simulink model "uzay_vektor"  (R2019b)
settings: Solver=ode1  StartTime=0.0  StopTime=0.02  FixedStep=1e-6  RelTol=1e-3
values from neighbouring files (symbols this model uses):
  m = 0.90    (= 0.9)    [uzay_vektor_parametreleri.m]
  Ts = 1/5000    (= 0.0002)    [uzay_vektor_parametreleri.m]
  Vdc = 250    [uzay_vektor_parametreleri.m]
  w = 2*pi*50    (= 314.159265359)    [uzay_vektor_parametreleri.m]
libraries: powerlib x20, simulink x12
settings Model: Creator=Monster  LastModifiedBy=Monster

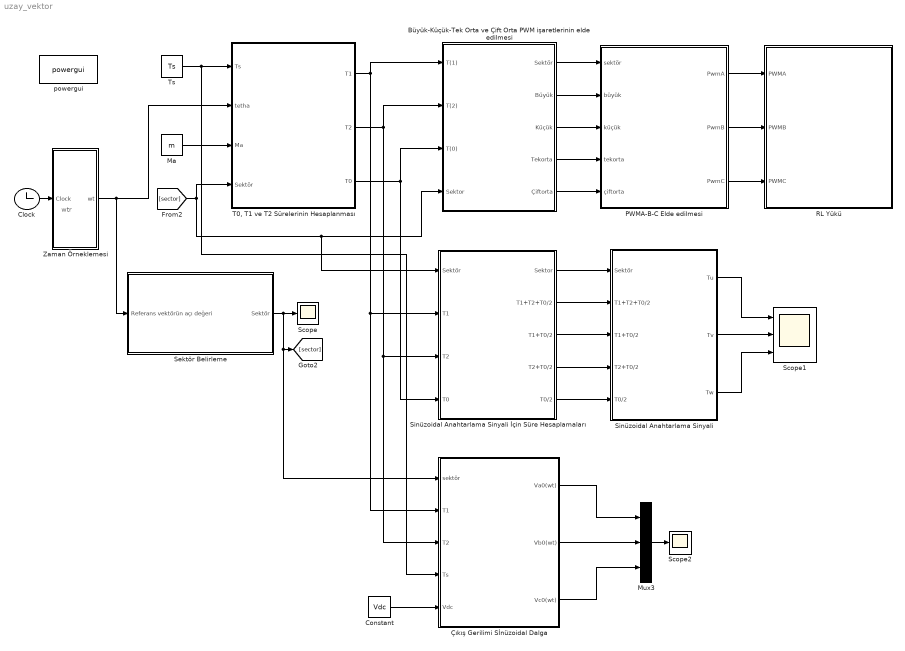
== system uzay_vektor ==
  note: wtr
  " Büyük-Küçük-Tek Orta ve Çift Orta PWM işaretlerinin elde edilmesi" : Subsystem
  " Clock" : Clock
  " Ma" : Constant  Value=m
  " PWMA-B-C Elde edilmesi" : Subsystem
  " RL Yükü" : Subsystem
  " Sektör Belirleme" : Subsystem
  " Sinüzoidal Anahtarlama Sinyali" : Subsystem
  " Sinüzoidal Anahtarlama Sinyali İçin Süre Hesaplamaları" : Subsystem
  " T0, T1 ve T2 Sürelerinin Hesaplanması" : Subsystem
  " Ts" : Constant  Value=Ts
  " Zaman Örneklemesi" : Subsystem
  " Çıkış Gerilimi Sİnüzoidal Dalga" : Subsystem
  Constant : Constant  Value=Vdc
  Mux3 : Mux  Inputs=3
  Scope : Scope
  Scope1 : Scope  NumInputPorts=3
  Scope2 : Scope
  "powergui " : powerlib/powergui  Priority=1  SimulationMode=Continuous  SampleTime=50e-6  frequency=60  Iterations=50  frequencyindice=0  Pbase=100e6  ErrMax=1e-4  UnitsV=kV  UnitsW=MW  buscounter=0  FunctionMessages=off  echomessages=off  EnableUseOfTLC=off  CurrentSourceSwitches=off  DisableSnubberDevices=off  DisableRonSwitches=off  DisableVfSwitches=off  DisplayEquations=off  AutomaticDiscreteSolvers=off  SolverType=Tustin/Backward Euler (TBE)  Interpol=off  ExternalGateDelay=off  methode=off  Ts=100  x0status=blocks  SPID=on  SwTol=0  HookPort=off  NonlinearTolerance=1e-4  nMaxIteration=100  ContinueOnMaxIteration=off  RestoreLinks=warning  ResistiveCurrentMeasurement=off  Frange=[0:2:500]  Ylog=off  Xlog=on  ShowGrid=off  save=off  variable=ZData  structure=0  ZoomFFT=off  StartTime=0.0  cycles=1  DisplayStyle=1  fundamental=60  FreqAxis=off  MaxFrequency=1000  frequencyindicesteady=1  RmsSteady=1  display=off
      settings: SourceProductName=Simscape Electrical
  wires:
  " Sektör Belirleme"/1(Sektör) -> " Çıkış Gerilimi Sİnüzoidal Dalga"/1("sektör "), [sector], Scope/1
  " Ts"/1 -> " Çıkış Gerilimi Sİnüzoidal Dalga"/4(Ts), " T0, T1 ve T2 Sürelerinin Hesaplanması"/1(Ts)
  [sector] -> " Sinüzoidal Anahtarlama Sinyali İçin Süre Hesaplamaları"/1(Sektör), " Büyük-Küçük-Tek Orta ve Çift Orta PWM işaretlerinin elde edilmesi"/4("Sektor "), " T0, T1 ve T2 Sürelerinin Hesaplanması"/4(Sektör)
  " Zaman Örneklemesi"/1("wt ") -> " Sektör Belirleme"/1(" Referans vektörün açı değeri"), " T0, T1 ve T2 Sürelerinin Hesaplanması"/2(tetha)
  " Clock"/1 -> " Zaman Örneklemesi"/1(Clock)
  " Ma"/1 -> " T0, T1 ve T2 Sürelerinin Hesaplanması"/3(Ma)
  " Büyük-Küçük-Tek Orta ve Çift Orta PWM işaretlerinin elde edilmesi"/1(Sektör) -> " PWMA-B-C Elde edilmesi"/1(sektör)
  " Büyük-Küçük-Tek Orta ve Çift Orta PWM işaretlerinin elde edilmesi"/2(Büyük) -> " PWMA-B-C Elde edilmesi"/2(büyük)
  " Büyük-Küçük-Tek Orta ve Çift Orta PWM işaretlerinin elde edilmesi"/3(Küçük) -> " PWMA-B-C Elde edilmesi"/3(küçük)
  " Büyük-Küçük-Tek Orta ve Çift Orta PWM işaretlerinin elde edilmesi"/4(Tekorta) -> " PWMA-B-C Elde edilmesi"/4(tekorta)
  " Büyük-Küçük-Tek Orta ve Çift Orta PWM işaretlerinin elde edilmesi"/5(Çiftorta) -> " PWMA-B-C Elde edilmesi"/5(çiftorta)
  " T0, T1 ve T2 Sürelerinin Hesaplanması"/3(T0) -> " Büyük-Küçük-Tek Orta ve Çift Orta PWM işaretlerinin elde edilmesi"/3(T(0)), " Sinüzoidal Anahtarlama Sinyali İçin Süre Hesaplamaları"/4(T0)
  " T0, T1 ve T2 Sürelerinin Hesaplanması"/2(T2) -> " Çıkış Gerilimi Sİnüzoidal Dalga"/3(T2), " Sinüzoidal Anahtarlama Sinyali İçin Süre Hesaplamaları"/3(T2), " Büyük-Küçük-Tek Orta ve Çift Orta PWM işaretlerinin elde edilmesi"/2(T(2))
  " T0, T1 ve T2 Sürelerinin Hesaplanması"/1(T1) -> " Çıkış Gerilimi Sİnüzoidal Dalga"/2(T1), " Sinüzoidal Anahtarlama Sinyali İçin Süre Hesaplamaları"/2(T1), " Büyük-Küçük-Tek Orta ve Çift Orta PWM işaretlerinin elde edilmesi"/1(T(1))
  " Sinüzoidal Anahtarlama Sinyali İçin Süre Hesaplamaları"/1(Sektor) -> " Sinüzoidal Anahtarlama Sinyali"/1(" Sektör")
  " Sinüzoidal Anahtarlama Sinyali İçin Süre Hesaplamaları"/2(T1+T2+T0/2) -> " Sinüzoidal Anahtarlama Sinyali"/2(" T1+T2+T0/2")
  " Sinüzoidal Anahtarlama Sinyali İçin Süre Hesaplamaları"/3(T1+T0/2) -> " Sinüzoidal Anahtarlama Sinyali"/3(" T1+T0/2")
  " Sinüzoidal Anahtarlama Sinyali İçin Süre Hesaplamaları"/4(T2+T0/2) -> " Sinüzoidal Anahtarlama Sinyali"/4(" T2+T0/2")
  " Sinüzoidal Anahtarlama Sinyali İçin Süre Hesaplamaları"/5(T0/2) -> " Sinüzoidal Anahtarlama Sinyali"/5(" T0/2")
  " Sinüzoidal Anahtarlama Sinyali"/2(" Tv") -> Scope1/2
  " Sinüzoidal Anahtarlama Sinyali"/1(" Tu") -> Scope1/1
  " Sinüzoidal Anahtarlama Sinyali"/3(" Tw") -> Scope1/3
  " PWMA-B-C Elde edilmesi"/1("PwmA ") -> " RL Yükü"/1(PWMA)
  " PWMA-B-C Elde edilmesi"/2("PwmB ") -> " RL Yükü"/2(PWMB)
  " PWMA-B-C Elde edilmesi"/3(PwmC) -> " RL Yükü"/3(PWMC)
  Mux3/1 -> Scope2/1
  " Çıkış Gerilimi Sİnüzoidal Dalga"/3(Vc0(wt)) -> Mux3/3
  " Çıkış Gerilimi Sİnüzoidal Dalga"/1(Va0(wt)) -> Mux3/1
  " Çıkış Gerilimi Sİnüzoidal Dalga"/2(Vb0(wt)) -> Mux3/2
  Constant/1 -> " Çıkış Gerilimi Sİnüzoidal Dalga"/5(Vdc)

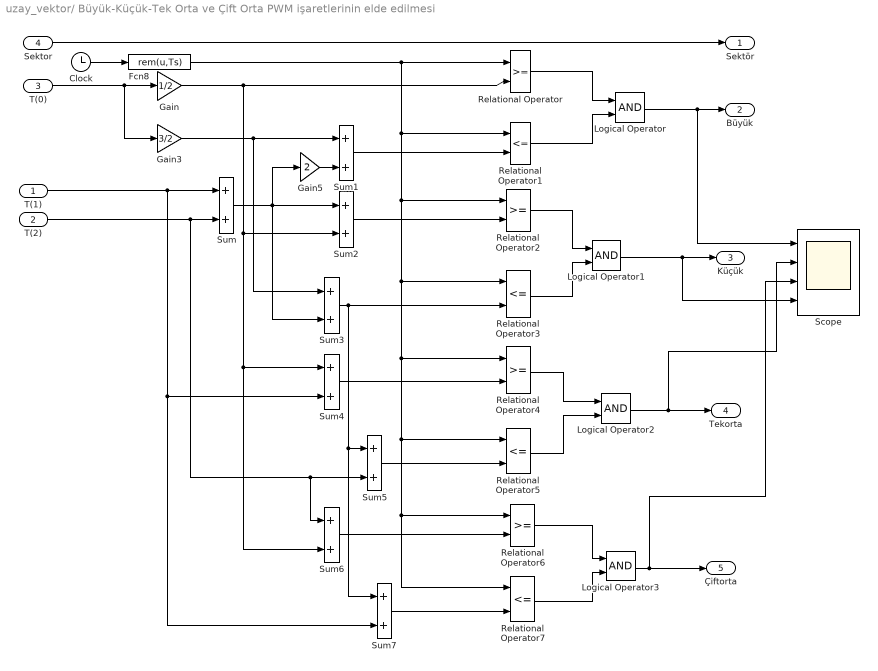
== system uzay_vektor/ Büyük-Küçük-Tek Orta ve Çift Orta PWM işaretlerinin elde edilmesi ==
  T(1) : Inport
  T(2) : Inport  Port=2
  T(0) : Inport  Port=3
  "Sektor " : Inport  Port=4
  Clock : Clock
  Fcn8 : Fcn  Expr=rem(u,Ts)
  Gain : Gain  Gain=1/2  SaturateOnIntegerOverflow=on  OutDataTypeStr=Inherit: Same as input  ParamDataTypeStr=Inherit: Same as input
  Gain3 : Gain  Gain=3/2  SaturateOnIntegerOverflow=on  OutDataTypeStr=Inherit: Same as input  ParamDataTypeStr=Inherit: Same as input
  Gain5 : Gain  Gain=2  SaturateOnIntegerOverflow=on  OutDataTypeStr=Inherit: Same as input  ParamDataTypeStr=Inherit: Same as input
  Logical Operator{,1..3} (4 alike) : Logic  AllPortsSameDT=off
  Relational Operator{,2,4,6} (4 alike) : RelationalOperator  RndMeth=Nearest
  Relational Operator{1,3,5,7} (4 alike) : RelationalOperator  Operator=<=  RndMeth=Nearest
  Scope : Scope  NumInputPorts=4
  Sum{,1..7} (8 alike) : Sum  SaturateOnIntegerOverflow=on
  Sektör : Outport
  Büyük : Outport  Port=2
  Küçük : Outport  Port=3
  Tekorta : Outport  Port=4
  Çiftorta : Outport  Port=5
  wires:
  Sum7/1 -> Relational Operator7/2
  Sum6/1 -> Relational Operator6/2
  Sum5/1 -> Relational Operator5/2
  Sum2/1 -> Relational Operator2/2
  Gain5/1 -> Sum1/2
  Gain3/1 -> Sum3/1, Sum1/1
  Sum/1 -> Sum3/2, Sum2/1, Gain5/1
  Clock/1 -> Fcn8/1
  Fcn8/1 -> Relational Operator/1, Relational Operator1/1, Relational Operator2/1, Relational Operator3/1, Relational Operator4/1, Relational Operator5/1, Relational Operator6/1, Relational Operator7/1
  T(0)/1 -> Gain3/1, Gain/1
  Gain/1 -> Relational Operator/2, Sum6/2, Sum4/1, Sum2/2
  T(1)/1 -> Sum7/2, Sum4/2, Sum/1
  T(2)/1 -> Sum6/1, Sum5/2, Sum/2
  Sum1/1 -> Relational Operator1/2
  Relational Operator/1 -> Logical Operator/1
  Relational Operator1/1 -> Logical Operator/2
  Logical Operator/1 -> Büyük/1, Scope/1
  Relational Operator2/1 -> Logical Operator1/1
  Relational Operator3/1 -> Logical Operator1/2
  Sum3/1 -> Sum7/1, Sum5/1, Relational Operator3/2
  Logical Operator1/1 -> Küçük/1, Scope/4
  Sum4/1 -> Relational Operator4/2
  Relational Operator4/1 -> Logical Operator2/1
  Relational Operator5/1 -> Logical Operator2/2
  Logical Operator2/1 -> Tekorta/1, Scope/2
  Relational Operator6/1 -> Logical Operator3/1
  Relational Operator7/1 -> Logical Operator3/2
  Logical Operator3/1 -> Çiftorta/1, Scope/3
  "Sektor "/1 -> Sektör/1

== system uzay_vektor/ PWMA-B-C Elde edilmesi ==
  sektör : Inport
  büyük : Inport  Port=2
  küçük : Inport  Port=3
  tekorta : Inport  Port=4
  çiftorta : Inport  Port=5
  PWMA-B-C : Scope  NumInputPorts=3
  Subsystem1 : Subsystem
  Subsystem2 : Subsystem
  Subsystem3 : Subsystem
  "PwmA " : Outport
  "PwmB " : Outport  Port=2
  PwmC : Outport  Port=3
  wires:
  sektör/1 -> Subsystem3/1(sektör), Subsystem1/1(sektör), Subsystem2/1(sektör)
  büyük/1 -> Subsystem3/2(Büyük), Subsystem1/2(Büyük), Subsystem2/2(Büyük)
  küçük/1 -> Subsystem3/3(Küçük), Subsystem1/3(Küçük), Subsystem2/3(Küçük)
  tekorta/1 -> Subsystem3/4(Tekorta), Subsystem1/4(Tekorta), Subsystem2/4(Tekorta)
  çiftorta/1 -> Subsystem3/5(çiftorta), Subsystem1/5(çiftorta), Subsystem2/5(çiftorta)
  Subsystem2/1(pwma) -> "PwmA "/1, PWMA-B-C/1
  Subsystem3/1(pwmc) -> PWMA-B-C/3, PwmC/1
  Subsystem1/1(pwmb) -> "PwmB "/1, PWMA-B-C/2

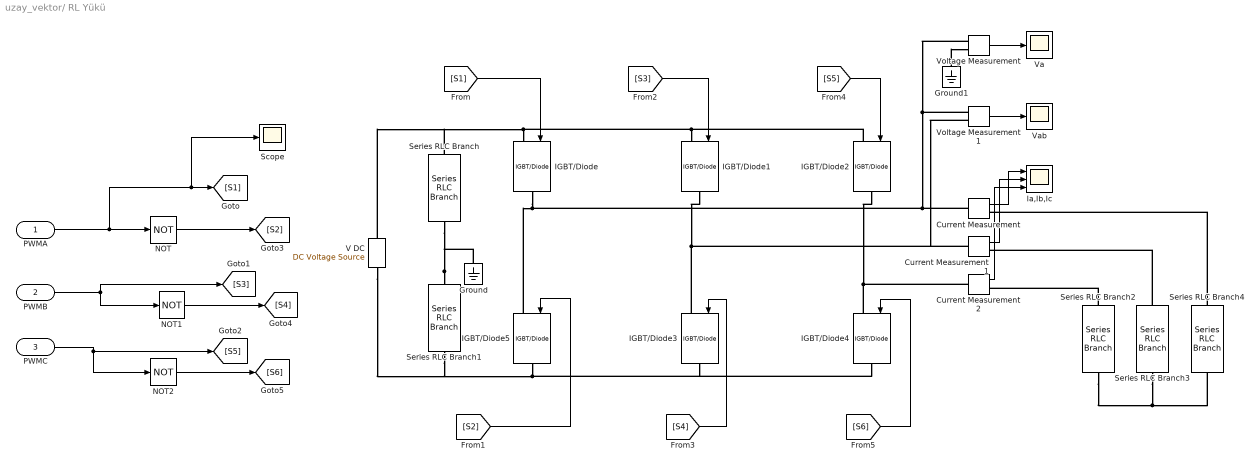
== system uzay_vektor/ RL Yükü ==
  PWMA : Inport
  PWMB : Inport  Port=2
  PWMC : Inport  Port=3
  " V DC" : powerlib/Electrical Sources/DC Voltage Source  Amplitude=Vdc  Measurements=None
      settings: SourceProductName=Simscape Electrical
  Current Measurement : powerlib/Measurements/Current Measurement  PhasorSimulation=off  OutputType=Complex  PSBequivalent=0
      settings: SourceProductName=Simscape Electrical
  Current Measurement1 : powerlib/Measurements/Current Measurement  PhasorSimulation=off  OutputType=Complex  PSBequivalent=0
      settings: SourceProductName=Simscape Electrical
  Current Measurement2 : powerlib/Measurements/Current Measurement  PhasorSimulation=off  OutputType=Complex  PSBequivalent=0
      settings: SourceProductName=Simscape Electrical
  Ground : powerlib/Elements/Ground  LConnTagsString=a
      settings: SourceProductName=Simscape Electrical
  Ground1 : powerlib/Elements/Ground  LConnTagsString=a
      settings: SourceProductName=Simscape Electrical
  "IGBT/Diode " : powerlib/Power Electronics/IGBT//Diode  Ron=1e-3  Rs=1e5  Cs=inf  Measurements=off
      settings: SourceProductName=Simscape Electrical
  IGBT/Diode{1..5} (5 alike) : powerlib/Power Electronics/IGBT//Diode  Ron=1e-3  Rs=1e5  Cs=inf  Measurements=off
      settings: SourceProductName=Simscape Electrical
  Ia,Ib,Ic : Scope  NumInputPorts=3
  "NOT " : Logic  Operator=NOT  IconShape=distinctive  AllPortsSameDT=off  OutDataTypeStr=boolean
  NOT1 : Logic  Operator=NOT  IconShape=distinctive  AllPortsSameDT=off  OutDataTypeStr=boolean
  NOT2 : Logic  Operator=NOT  IconShape=distinctive  AllPortsSameDT=off  OutDataTypeStr=boolean
  Scope : Scope
  Series RLC Branch : powerlib/Elements/Series RLC Branch  LConnTagsString=__new0  RConnTagsString=__new0  BranchType=RC  Resistance=0.01  Inductance=5000e-6  SetiL0=off  InitialCurrent=0  Capacitance=5000e-6  Setx0=off  InitialVoltage=0  Measurements=None
      settings: SourceProductName=Simscape Electrical
  Series RLC Branch1 : powerlib/Elements/Series RLC Branch  LConnTagsString=__new0  RConnTagsString=__new0  BranchType=RC  Resistance=0.01  Inductance=5000e-6  SetiL0=off  InitialCurrent=0  Capacitance=5000e-6  Setx0=off  InitialVoltage=0  Measurements=None
      settings: SourceProductName=Simscape Electrical
  Series RLC Branch2 : powerlib/Elements/Series RLC Branch  LConnTagsString=__new0  RConnTagsString=__new0  BranchType=RL  Resistance=30  Inductance=30e-3  SetiL0=off  InitialCurrent=0  Capacitance=30e-3  Setx0=off  InitialVoltage=0  Measurements=None
      settings: SourceProductName=Simscape Electrical
  Series RLC Branch3 : powerlib/Elements/Series RLC Branch  LConnTagsString=__new0  RConnTagsString=__new0  BranchType=RL  Resistance=30  Inductance=30e-3  SetiL0=off  InitialCurrent=0  Capacitance=30e-3  Setx0=off  InitialVoltage=0  Measurements=None
      settings: SourceProductName=Simscape Electrical
  Series RLC Branch4 : powerlib/Elements/Series RLC Branch  LConnTagsString=__new0  RConnTagsString=__new0  BranchType=RL  Resistance=30  Inductance=30e-3  SetiL0=off  InitialCurrent=0  Capacitance=30e-3  Setx0=off  InitialVoltage=0  Measurements=None
      settings: SourceProductName=Simscape Electrical
  Va : Scope
  Vab : Scope
  Voltage Measurement : powerlib/Measurements/Voltage Measurement  PhasorSimulation=off  OutputType=Complex  PSBequivalent=0
      settings: SourceProductName=Simscape Electrical
  Voltage Measurement1 : powerlib/Measurements/Voltage Measurement  PhasorSimulation=off  OutputType=Complex  PSBequivalent=0
      settings: SourceProductName=Simscape Electrical
  wires:
  [S4] -> IGBT/Diode3/1
  Current Measurement2/1 -> Ia,Ib,Ic/3
  Current Measurement/1 -> Ia,Ib,Ic/1
  Current Measurement1/1 -> Ia,Ib,Ic/2
  Voltage Measurement1/1 -> Vab/1
  Voltage Measurement/1 -> Va/1
  PWMA/1 -> "NOT "/1, Scope/1, [S1]
  [S5] -> IGBT/Diode2/1
  "NOT "/1 -> [S2]
  NOT2/1 -> [S6]
  PWMC/1 -> NOT2/1, [S5]
  [S1] -> "IGBT/Diode "/1
  NOT1/1 -> [S4]
  [S3] -> IGBT/Diode1/1
  [S2] -> IGBT/Diode5/1
  [S6] -> IGBT/Diode4/1
  PWMB/1 -> NOT1/1, [S3]
  connections:
  Voltage Measurement1/LConn1 -- Current Measurement/LConn1 -- IGBT/Diode5/LConn1 -- "IGBT/Diode "/RConn1 -- Voltage Measurement/LConn1
  IGBT/Diode2/RConn1 -- Current Measurement2/LConn1 -- IGBT/Diode4/LConn1
  IGBT/Diode5/RConn1 -- " V DC"/LConn1 -- Series RLC Branch1/RConn1 -- IGBT/Diode4/RConn1 -- IGBT/Diode3/RConn1
  Series RLC Branch3/RConn1 -- Series RLC Branch2/RConn1 -- Series RLC Branch4/RConn1
  IGBT/Diode1/RConn1 -- Current Measurement1/LConn1 -- Voltage Measurement1/LConn2 -- IGBT/Diode3/LConn1
  Series RLC Branch1/LConn1 -- Ground/LConn1 -- Series RLC Branch/RConn1
  IGBT/Diode1/LConn1 -- " V DC"/RConn1 -- Series RLC Branch/LConn1 -- "IGBT/Diode "/LConn1 -- IGBT/Diode2/LConn1
  Series RLC Branch2/LConn1 -- Current Measurement2/RConn1
  Ground1/LConn1 -- Voltage Measurement/LConn2
  Series RLC Branch4/LConn1 -- Current Measurement/RConn1
  Series RLC Branch3/LConn1 -- Current Measurement1/RConn1

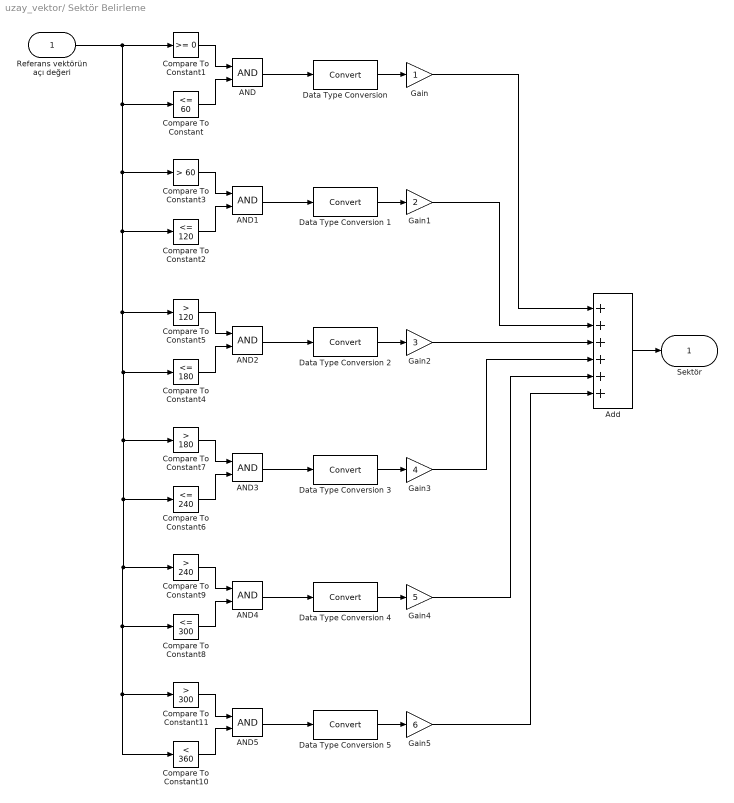
== system uzay_vektor/ Sektör Belirleme ==
  " Referans vektörün açı değeri" : Inport
  AND{,1..5} (6 alike) : Logic  AllPortsSameDT=off  OutDataTypeStr=boolean
  Add : Sum  Inputs=++++++
  Compare To Constant : simulink/Logic and Bit Operations/Compare To Constant  relop=<=  const=60  OutDataTypeStr=boolean
  Compare To Constant1 : simulink/Logic and Bit Operations/Compare To Constant  relop=>=  const=0  OutDataTypeStr=boolean
  Compare To Constant10 : simulink/Logic and Bit Operations/Compare To Constant  relop=<  const=360  OutDataTypeStr=boolean
  Compare To Constant11 : simulink/Logic and Bit Operations/Compare To Constant  relop=>  const=300  OutDataTypeStr=boolean
  Compare To Constant2 : simulink/Logic and Bit Operations/Compare To Constant  relop=<=  const=120  OutDataTypeStr=boolean
  Compare To Constant3 : simulink/Logic and Bit Operations/Compare To Constant  relop=>  const=60  OutDataTypeStr=boolean
  Compare To Constant4 : simulink/Logic and Bit Operations/Compare To Constant  relop=<=  const=180  OutDataTypeStr=boolean
  Compare To Constant5 : simulink/Logic and Bit Operations/Compare To Constant  relop=>  const=120  OutDataTypeStr=boolean
  Compare To Constant6 : simulink/Logic and Bit Operations/Compare To Constant  relop=<=  const=240  OutDataTypeStr=boolean
  Compare To Constant7 : simulink/Logic and Bit Operations/Compare To Constant  relop=>  const=180  OutDataTypeStr=boolean
  Compare To Constant8 : simulink/Logic and Bit Operations/Compare To Constant  relop=<=  const=300  OutDataTypeStr=boolean
  Compare To Constant9 : simulink/Logic and Bit Operations/Compare To Constant  relop=>  const=240  OutDataTypeStr=boolean
  Data Type Conversion {,1..5} (6 alike) : DataTypeConversion
  Gain : Gain
  Gain1 : Gain  Gain=2
  Gain2 : Gain  Gain=3
  Gain3 : Gain  Gain=4
  Gain4 : Gain  Gain=5
  Gain5 : Gain  Gain=6
  Sektör : Outport
  wires:
  Compare To Constant1/1 -> AND/1
  Compare To Constant/1 -> AND/2
  AND/1 -> "Data Type Conversion "/1
  "Data Type Conversion "/1 -> Gain/1
  Data Type Conversion 1/1 -> Gain1/1
  AND1/1 -> Data Type Conversion 1/1
  Compare To Constant2/1 -> AND1/2
  Compare To Constant3/1 -> AND1/1
  Compare To Constant7/1 -> AND3/1
  Compare To Constant6/1 -> AND3/2
  AND3/1 -> Data Type Conversion 3/1
  Data Type Conversion 3/1 -> Gain3/1
  Data Type Conversion 2/1 -> Gain2/1
  AND2/1 -> Data Type Conversion 2/1
  Compare To Constant4/1 -> AND2/2
  Compare To Constant5/1 -> AND2/1
  Compare To Constant9/1 -> AND4/1
  Compare To Constant8/1 -> AND4/2
  AND4/1 -> Data Type Conversion 4/1
  Data Type Conversion 4/1 -> Gain4/1
  Data Type Conversion 5/1 -> Gain5/1
  AND5/1 -> Data Type Conversion 5/1
  Compare To Constant10/1 -> AND5/2
  Compare To Constant11/1 -> AND5/1
  " Referans vektörün açı değeri"/1 -> Compare To Constant10/1, Compare To Constant11/1, Compare To Constant8/1, Compare To Constant9/1, Compare To Constant6/1, Compare To Constant7/1, Compare To Constant4/1, Compare To Constant5/1, Compare To Constant2/1, Compare To Constant3/1, Compare To Constant/1, Compare To Constant1/1
  Gain/1 -> Add/1
  Gain1/1 -> Add/2
  Gain2/1 -> Add/3
  Gain3/1 -> Add/4
  Gain4/1 -> Add/5
  Gain5/1 -> Add/6
  Add/1 -> Sektör/1

== system uzay_vektor/ Sinüzoidal Anahtarlama Sinyali ==
  " Sektör" : Inport
  " T1+T2+T0/2" : Inport  Port=2
  " T1+T0/2" : Inport  Port=3
  " T2+T0/2" : Inport  Port=4
  " T0/2" : Inport  Port=5
  S1 : MultiPortSwitch  DataPortOrder=Specify indices  Inputs=6  DataPortIndices={[1,6], 2,5,[3,4]}
  S3 : MultiPortSwitch  DataPortOrder=Specify indices  Inputs=6  DataPortIndices={ [2, 3], 4,1, [5, 6]}
  S5 : MultiPortSwitch  DataPortOrder=Specify indices  Inputs=6  DataPortIndices={ [4,5],6, 3, [1, 2]}
  " Tu" : Outport
  " Tv" : Outport  Port=2
  " Tw" : Outport  Port=3
  wires:
  S3/1 -> " Tv"/1
  S5/1 -> " Tw"/1
  S1/1 -> " Tu"/1
  " Sektör"/1 -> S5/1, S3/1, S1/1
  " T2+T0/2"/1 -> S1/4, S5/4, S3/4
  " T1+T0/2"/1 -> S1/3, S5/3, S3/3
  " T1+T2+T0/2"/1 -> S1/2, S5/2, S3/2
  " T0/2"/1 -> S1/5, S5/5, S3/5

== system uzay_vektor/ Sinüzoidal Anahtarlama Sinyali İçin Süre Hesaplamaları ==
  Sektör : Inport
  T1 : Inport  Port=2
  T2 : Inport  Port=3
  T0 : Inport  Port=4
  Add : Sum
  Add1 : Sum
  Gain : Gain  Gain=1/2
  TOPLAMA : Sum  Inputs=+++
  Sektor : Outport
  T1+T2+T0/2 : Outport  Port=2
  T1+T0/2 : Outport  Port=3
  T2+T0/2 : Outport  Port=4
  T0/2 : Outport  Port=5
  wires:
  T0/1 -> Gain/1
  T1/1 -> Add/1, TOPLAMA/1
  T2/1 -> TOPLAMA/2, Add1/1
  Gain/1 -> T0/2/1, Add1/2, Add/2, TOPLAMA/3
  TOPLAMA/1 -> T1+T2+T0/2/1
  Add/1 -> T1+T0/2/1
  Add1/1 -> T2+T0/2/1
  Sektör/1 -> Sektor/1

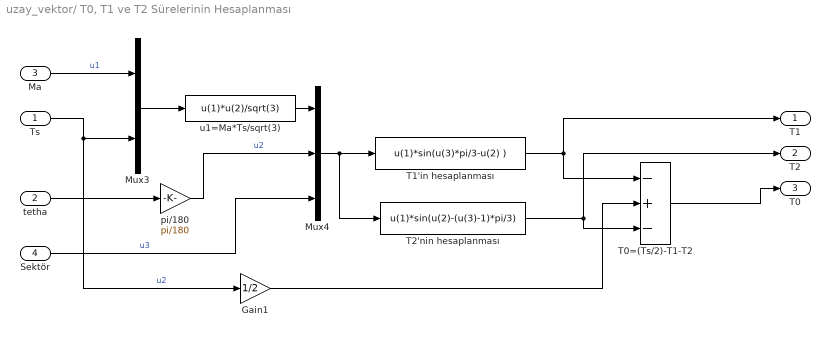
== system uzay_vektor/ T0, T1 ve T2 Sürelerinin Hesaplanması ==
  Ts : Inport
  tetha : Inport  Port=2
  Ma : Inport  Port=3
  Sektör : Inport  Port=4
  Gain1 : Gain  Gain=1/2
  Mux3 : Mux  Inputs=2
  Mux4 : Mux  Inputs=3
  T0=(Ts/2)-T1-T2 : Sum  Inputs=-+-
  T1'in hesaplanması : Fcn  Expr=u(1)*sin(u(3)*pi/3-u(2) )
  T2'nin hesaplanması : Fcn  Expr=u(1)*sin(u(2)-(u(3)-1)*pi/3)
  pi/180 : Gain  Gain=pi/180
  u1=Ma*Ts/sqrt(3) : Fcn  Expr=u(1)*u(2)/sqrt(3)
  T1 : Outport
  T2 : Outport  Port=2
  T0 : Outport  Port=3
  wires:
  T1'in hesaplanması/1 -> T0=(Ts/2)-T1-T2/1, T1/1
  T2'nin hesaplanması/1 -> T0=(Ts/2)-T1-T2/3, T2/1
  Mux3/1 -> u1=Ma*Ts/sqrt(3)/1
  Mux4/1 -> T2'nin hesaplanması/1, T1'in hesaplanması/1
  u1=Ma*Ts/sqrt(3)/1 -> Mux4/1
  Ts/1 -> Gain1/1, Mux3/2  "u2"
  Sektör/1 -> Mux4/3  "u3"
  Gain1/1 -> T0=(Ts/2)-T1-T2/2
  tetha/1 -> pi/180/1
  pi/180/1 -> Mux4/2  "u2"
  Ma/1 -> Mux3/1  "u1"
  T0=(Ts/2)-T1-T2/1 -> T0/1

== system uzay_vektor/ Zaman Örneklemesi ==
  Clock : Inport
  2*pi*50 : Constant  Value=w
  Constant2 : Constant  Value=2*pi
  Constant3 : Constant  Value=180/pi
  Math Function : Math  Operator=mod  SaturateOnIntegerOverflow=on
  Product1 : Product
  Product2 : Product  SaturateOnIntegerOverflow=on  OutDataTypeStr=Inherit: Same as first input
  "Scope " : Scope
  "Zero-Order Hold " : ZeroOrderHold  SampleTime=Ts
  "wt " : Outport
  wires:
  Product1/1 -> "Scope "/1, "wt "/1
  "Zero-Order Hold "/1 -> Product2/1
  2*pi*50/1 -> Product2/2
  Clock/1 -> "Zero-Order Hold "/1
  Constant3/1 -> Product1/2
  Constant2/1 -> Math Function/2
  Product2/1 -> Math Function/1
  Math Function/1 -> Product1/1

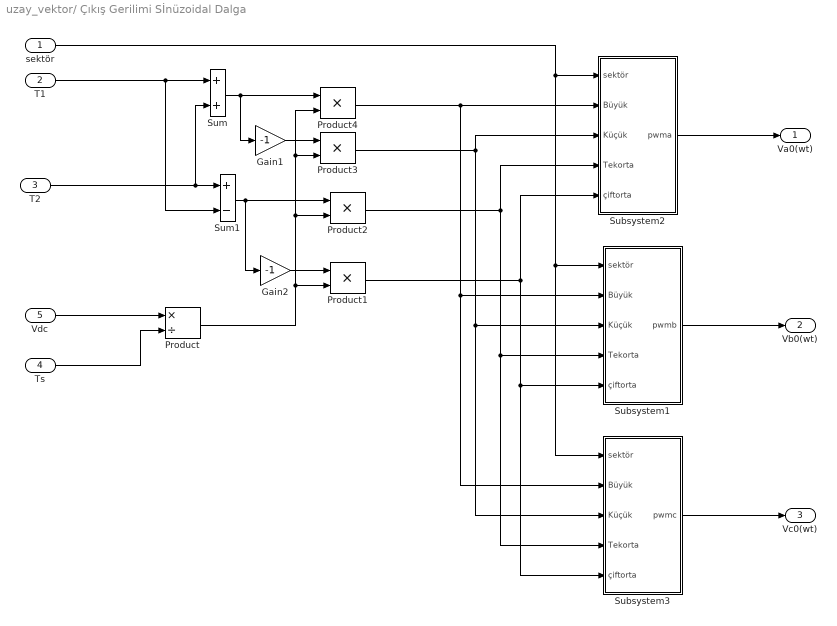
== system uzay_vektor/ Çıkış Gerilimi Sİnüzoidal Dalga ==
  "sektör " : Inport
  T1 : Inport  Port=2
  T2 : Inport  Port=3
  Ts : Inport  Port=4
  Vdc : Inport  Port=5
  Gain1 : Gain  Gain=-1  SaturateOnIntegerOverflow=on  OutDataTypeStr=Inherit: Same as input  ParamDataTypeStr=Inherit: Same as input
  Gain2 : Gain  Gain=-1  SaturateOnIntegerOverflow=on  OutDataTypeStr=Inherit: Same as input  ParamDataTypeStr=Inherit: Same as input
  Product : Product  Inputs=*/  SaturateOnIntegerOverflow=on  OutDataTypeStr=Inherit: Same as first input
  Product{1..4} (4 alike) : Product  SaturateOnIntegerOverflow=on  OutDataTypeStr=Inherit: Same as first input
  Subsystem1 : Subsystem
  Subsystem2 : Subsystem
  Subsystem3 : Subsystem
  Sum : Sum  SaturateOnIntegerOverflow=on
  Sum1 : Sum  Inputs=+-  SaturateOnIntegerOverflow=on
  Va0(wt) : Outport
  Vb0(wt) : Outport  Port=2
  Vc0(wt) : Outport  Port=3
  wires:
  Subsystem2/1(pwma) -> Va0(wt)/1
  Subsystem1/1(pwmb) -> Vb0(wt)/1
  Subsystem3/1(pwmc) -> Vc0(wt)/1
  "sektör "/1 -> Subsystem2/1(sektör), Subsystem1/1(sektör), Subsystem3/1(sektör)
  T1/1 -> Sum/1, Sum1/2
  T2/1 -> Sum/2, Sum1/1
  Sum/1 -> Product4/1, Gain1/1
  Sum1/1 -> Gain2/1, Product2/1
  Ts/1 -> Product/2
  Vdc/1 -> Product/1
  Product/1 -> Product1/2, Product2/2, Product3/2, Product4/2
  Gain1/1 -> Product3/1
  Product4/1 -> Subsystem2/2(Büyük), Subsystem1/2(Büyük), Subsystem3/2(Büyük)
  Product3/1 -> Subsystem2/3(Küçük), Subsystem1/3(Küçük), Subsystem3/3(Küçük)
  Gain2/1 -> Product1/1
  Product2/1 -> Subsystem2/4(Tekorta), Subsystem1/4(Tekorta), Subsystem3/4(Tekorta)
  Product1/1 -> Subsystem2/5(çiftorta), Subsystem1/5(çiftorta), Subsystem3/5(çiftorta)

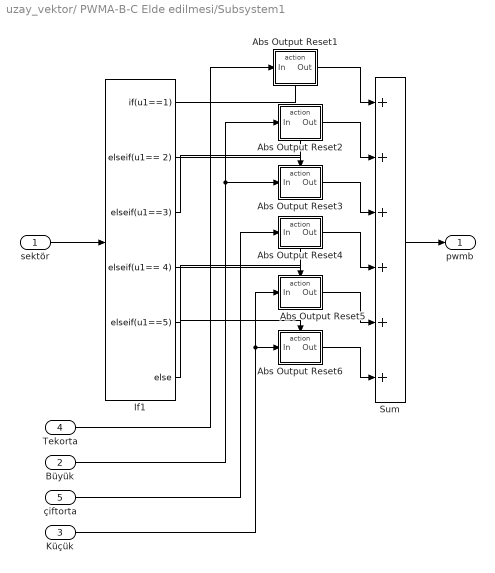
== system uzay_vektor/ PWMA-B-C Elde edilmesi/Subsystem1 ==
  sektör : Inport
  Büyük : Inport  Port=2
  Küçük : Inport  Port=3
  Tekorta : Inport  Port=4
  çiftorta : Inport  Port=5
  Abs Output Reset1 : Subsystem  TreatAsAtomicUnit=on
  Abs Output Reset2 : Subsystem  TreatAsAtomicUnit=on
  Abs Output Reset3 : Subsystem  TreatAsAtomicUnit=on
  Abs Output Reset4 : Subsystem  TreatAsAtomicUnit=on
  Abs Output Reset5 : Subsystem  TreatAsAtomicUnit=on
  Abs Output Reset6 : Subsystem  TreatAsAtomicUnit=on
  If1 : If  IfExpression=u1==1  ElseIfExpressions=u1== 2,u1==3 , u1== 4,u1==5
  Sum : Sum  Inputs=++++++  OutDataTypeStr=double  SaturateOnIntegerOverflow=on
  pwmb : Outport
  wires:
  Abs Output Reset1/1(Out) -> Sum/1
  Abs Output Reset2/1(Out) -> Sum/2
  Abs Output Reset3/1(Out) -> Sum/3
  Abs Output Reset4/1(Out) -> Sum/4
  Abs Output Reset5/1(Out) -> Sum/5
  Abs Output Reset6/1(Out) -> Sum/6
  sektör/1 -> If1/1
  Sum/1 -> pwmb/1
  If1/1 -> Abs Output Reset1/Action
  If1/2 -> Abs Output Reset2/Action
  If1/3 -> Abs Output Reset3/Action
  If1/4 -> Abs Output Reset4/Action
  If1/5 -> Abs Output Reset5/Action
  If1/6 -> Abs Output Reset6/Action
  Tekorta/1 -> Abs Output Reset1/1(In)
  Büyük/1 -> Abs Output Reset2/1(In), Abs Output Reset3/1(In)
  çiftorta/1 -> Abs Output Reset4/1(In)
  Küçük/1 -> Abs Output Reset5/1(In), Abs Output Reset6/1(In)

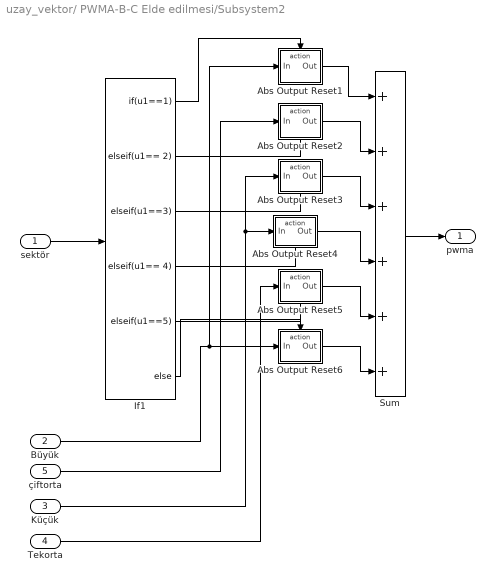
== system uzay_vektor/ PWMA-B-C Elde edilmesi/Subsystem2 ==
  sektör : Inport
  Büyük : Inport  Port=2
  Küçük : Inport  Port=3
  Tekorta : Inport  Port=4
  çiftorta : Inport  Port=5
  Abs Output Reset1 : Subsystem  TreatAsAtomicUnit=on
  Abs Output Reset2 : Subsystem  TreatAsAtomicUnit=on
  Abs Output Reset3 : Subsystem  TreatAsAtomicUnit=on
  Abs Output Reset4 : Subsystem  TreatAsAtomicUnit=on
  Abs Output Reset5 : Subsystem  TreatAsAtomicUnit=on
  Abs Output Reset6 : Subsystem  TreatAsAtomicUnit=on
  If1 : If  IfExpression=u1==1  ElseIfExpressions=u1== 2,u1==3 , u1== 4,u1==5
  Sum : Sum  Inputs=++++++  OutDataTypeStr=double  SaturateOnIntegerOverflow=on
  pwma : Outport
  wires:
  Sum/1 -> pwma/1
  sektör/1 -> If1/1
  Abs Output Reset6/1(Out) -> Sum/6
  Abs Output Reset5/1(Out) -> Sum/5
  Abs Output Reset4/1(Out) -> Sum/4
  Abs Output Reset3/1(Out) -> Sum/3
  Abs Output Reset2/1(Out) -> Sum/2
  Abs Output Reset1/1(Out) -> Sum/1
  If1/1 -> Abs Output Reset1/Action
  If1/2 -> Abs Output Reset2/Action
  If1/3 -> Abs Output Reset3/Action
  If1/4 -> Abs Output Reset4/Action
  If1/5 -> Abs Output Reset5/Action
  If1/6 -> Abs Output Reset6/Action
  Büyük/1 -> Abs Output Reset1/1(In), Abs Output Reset6/1(In)
  çiftorta/1 -> Abs Output Reset2/1(In)
  Küçük/1 -> Abs Output Reset3/1(In), Abs Output Reset4/1(In)
  Tekorta/1 -> Abs Output Reset5/1(In)

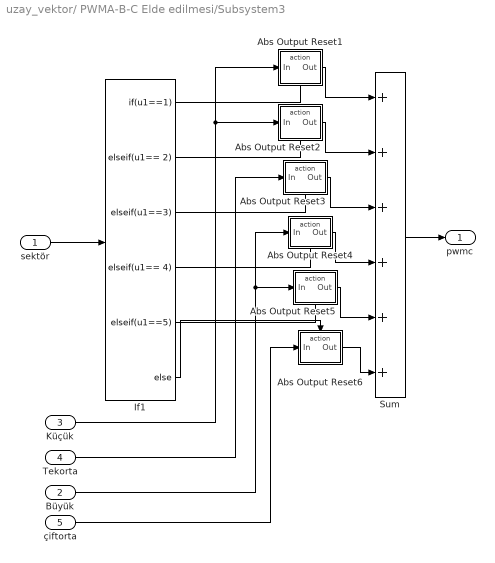
== system uzay_vektor/ PWMA-B-C Elde edilmesi/Subsystem3 ==
  sektör : Inport
  Büyük : Inport  Port=2
  Küçük : Inport  Port=3
  Tekorta : Inport  Port=4
  çiftorta : Inport  Port=5
  Abs Output Reset1 : Subsystem  TreatAsAtomicUnit=on
  Abs Output Reset2 : Subsystem  TreatAsAtomicUnit=on
  Abs Output Reset3 : Subsystem  TreatAsAtomicUnit=on
  Abs Output Reset4 : Subsystem  TreatAsAtomicUnit=on
  Abs Output Reset5 : Subsystem  TreatAsAtomicUnit=on
  Abs Output Reset6 : Subsystem  TreatAsAtomicUnit=on
  If1 : If  IfExpression=u1==1  ElseIfExpressions=u1== 2,u1==3 , u1== 4,u1==5
  Sum : Sum  Inputs=++++++  OutDataTypeStr=double  SaturateOnIntegerOverflow=on
  pwmc : Outport
  wires:
  Sum/1 -> pwmc/1
  sektör/1 -> If1/1
  Abs Output Reset6/1(Out) -> Sum/6
  Abs Output Reset5/1(Out) -> Sum/5
  Abs Output Reset4/1(Out) -> Sum/4
  Abs Output Reset3/1(Out) -> Sum/3
  Abs Output Reset2/1(Out) -> Sum/2
  Abs Output Reset1/1(Out) -> Sum/1
  If1/1 -> Abs Output Reset1/Action
  If1/2 -> Abs Output Reset2/Action
  If1/3 -> Abs Output Reset3/Action
  If1/4 -> Abs Output Reset4/Action
  If1/5 -> Abs Output Reset5/Action
  If1/6 -> Abs Output Reset6/Action
  Küçük/1 -> Abs Output Reset1/1(In), Abs Output Reset2/1(In)
  Tekorta/1 -> Abs Output Reset3/1(In)
  Büyük/1 -> Abs Output Reset4/1(In), Abs Output Reset5/1(In)
  çiftorta/1 -> Abs Output Reset6/1(In)

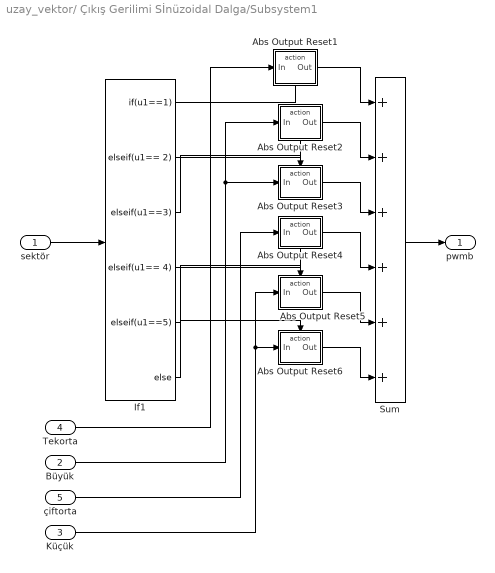
== system uzay_vektor/ Çıkış Gerilimi Sİnüzoidal Dalga/Subsystem1 ==
  sektör : Inport
  Büyük : Inport  Port=2
  Küçük : Inport  Port=3
  Tekorta : Inport  Port=4
  çiftorta : Inport  Port=5
  Abs Output Reset1 : Subsystem  TreatAsAtomicUnit=on
  Abs Output Reset2 : Subsystem  TreatAsAtomicUnit=on
  Abs Output Reset3 : Subsystem  TreatAsAtomicUnit=on
  Abs Output Reset4 : Subsystem  TreatAsAtomicUnit=on
  Abs Output Reset5 : Subsystem  TreatAsAtomicUnit=on
  Abs Output Reset6 : Subsystem  TreatAsAtomicUnit=on
  If1 : If  IfExpression=u1==1  ElseIfExpressions=u1== 2,u1==3 , u1== 4,u1==5
  Sum : Sum  Inputs=++++++  OutDataTypeStr=double  SaturateOnIntegerOverflow=on
  pwmb : Outport
  wires:
  Abs Output Reset1/1(Out) -> Sum/1
  Abs Output Reset2/1(Out) -> Sum/2
  Abs Output Reset3/1(Out) -> Sum/3
  Abs Output Reset4/1(Out) -> Sum/4
  Abs Output Reset5/1(Out) -> Sum/5
  Abs Output Reset6/1(Out) -> Sum/6
  sektör/1 -> If1/1
  Sum/1 -> pwmb/1
  If1/1 -> Abs Output Reset1/Action
  If1/2 -> Abs Output Reset2/Action
  If1/3 -> Abs Output Reset3/Action
  If1/4 -> Abs Output Reset4/Action
  If1/5 -> Abs Output Reset5/Action
  If1/6 -> Abs Output Reset6/Action
  Tekorta/1 -> Abs Output Reset1/1(In)
  Büyük/1 -> Abs Output Reset2/1(In), Abs Output Reset3/1(In)
  çiftorta/1 -> Abs Output Reset4/1(In)
  Küçük/1 -> Abs Output Reset5/1(In), Abs Output Reset6/1(In)

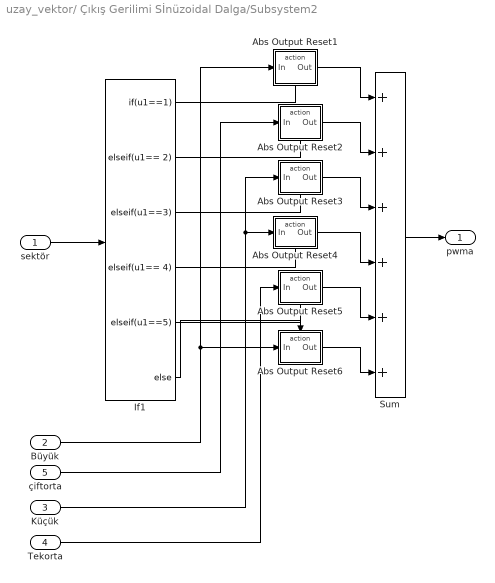
== system uzay_vektor/ Çıkış Gerilimi Sİnüzoidal Dalga/Subsystem2 ==
  sektör : Inport
  Büyük : Inport  Port=2
  Küçük : Inport  Port=3
  Tekorta : Inport  Port=4
  çiftorta : Inport  Port=5
  Abs Output Reset1 : Subsystem  TreatAsAtomicUnit=on
  Abs Output Reset2 : Subsystem  TreatAsAtomicUnit=on
  Abs Output Reset3 : Subsystem  TreatAsAtomicUnit=on
  Abs Output Reset4 : Subsystem  TreatAsAtomicUnit=on
  Abs Output Reset5 : Subsystem  TreatAsAtomicUnit=on
  Abs Output Reset6 : Subsystem  TreatAsAtomicUnit=on
  If1 : If  IfExpression=u1==1  ElseIfExpressions=u1== 2,u1==3 , u1== 4,u1==5
  Sum : Sum  Inputs=++++++  OutDataTypeStr=double  SaturateOnIntegerOverflow=on
  pwma : Outport
  wires:
  Sum/1 -> pwma/1
  sektör/1 -> If1/1
  Abs Output Reset6/1(Out) -> Sum/6
  Abs Output Reset5/1(Out) -> Sum/5
  Abs Output Reset4/1(Out) -> Sum/4
  Abs Output Reset3/1(Out) -> Sum/3
  Abs Output Reset2/1(Out) -> Sum/2
  Abs Output Reset1/1(Out) -> Sum/1
  If1/1 -> Abs Output Reset1/Action
  If1/2 -> Abs Output Reset2/Action
  If1/3 -> Abs Output Reset3/Action
  If1/4 -> Abs Output Reset4/Action
  If1/5 -> Abs Output Reset5/Action
  If1/6 -> Abs Output Reset6/Action
  Büyük/1 -> Abs Output Reset1/1(In), Abs Output Reset6/1(In)
  çiftorta/1 -> Abs Output Reset2/1(In)
  Küçük/1 -> Abs Output Reset3/1(In), Abs Output Reset4/1(In)
  Tekorta/1 -> Abs Output Reset5/1(In)

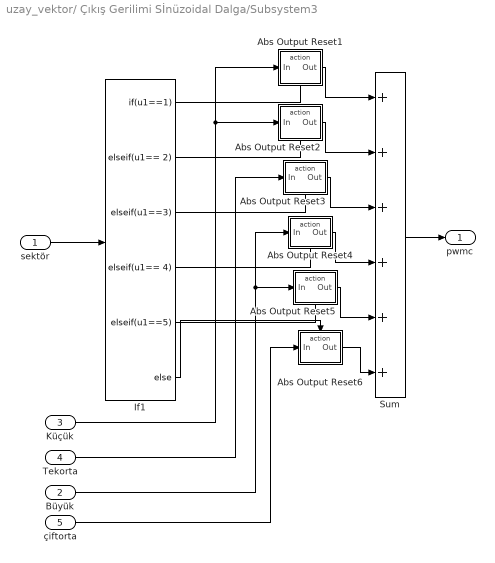
== system uzay_vektor/ Çıkış Gerilimi Sİnüzoidal Dalga/Subsystem3 ==
  sektör : Inport
  Büyük : Inport  Port=2
  Küçük : Inport  Port=3
  Tekorta : Inport  Port=4
  çiftorta : Inport  Port=5
  Abs Output Reset1 : Subsystem  TreatAsAtomicUnit=on
  Abs Output Reset2 : Subsystem  TreatAsAtomicUnit=on
  Abs Output Reset3 : Subsystem  TreatAsAtomicUnit=on
  Abs Output Reset4 : Subsystem  TreatAsAtomicUnit=on
  Abs Output Reset5 : Subsystem  TreatAsAtomicUnit=on
  Abs Output Reset6 : Subsystem  TreatAsAtomicUnit=on
  If1 : If  IfExpression=u1==1  ElseIfExpressions=u1== 2,u1==3 , u1== 4,u1==5
  Sum : Sum  Inputs=++++++  OutDataTypeStr=double  SaturateOnIntegerOverflow=on
  pwmc : Outport
  wires:
  Sum/1 -> pwmc/1
  sektör/1 -> If1/1
  Abs Output Reset6/1(Out) -> Sum/6
  Abs Output Reset5/1(Out) -> Sum/5
  Abs Output Reset4/1(Out) -> Sum/4
  Abs Output Reset3/1(Out) -> Sum/3
  Abs Output Reset2/1(Out) -> Sum/2
  Abs Output Reset1/1(Out) -> Sum/1
  If1/1 -> Abs Output Reset1/Action
  If1/2 -> Abs Output Reset2/Action
  If1/3 -> Abs Output Reset3/Action
  If1/4 -> Abs Output Reset4/Action
  If1/5 -> Abs Output Reset5/Action
  If1/6 -> Abs Output Reset6/Action
  Küçük/1 -> Abs Output Reset1/1(In), Abs Output Reset2/1(In)
  Tekorta/1 -> Abs Output Reset3/1(In)
  Büyük/1 -> Abs Output Reset4/1(In), Abs Output Reset5/1(In)
  çiftorta/1 -> Abs Output Reset6/1(In)

== system uzay_vektor/ PWMA-B-C Elde edilmesi/Subsystem1/Abs Output Reset1 ==
  In : Inport
  Action : ActionPort  ActionPortLabel=if(u1==1)
  Out : Outport  OutputWhenDisabled=reset  InitialOutput=0
  wires:
  In/1 -> Out/1

== system uzay_vektor/ PWMA-B-C Elde edilmesi/Subsystem1/Abs Output Reset2 ==
  In : Inport
  Action : ActionPort  ActionPortLabel=elseif(u1== 2)
  Out : Outport  OutputWhenDisabled=reset  InitialOutput=0
  wires:
  In/1 -> Out/1

== system uzay_vektor/ PWMA-B-C Elde edilmesi/Subsystem1/Abs Output Reset3 ==
  In : Inport
  Action : ActionPort  ActionPortLabel=elseif(u1==3 )
  Out : Outport  OutputWhenDisabled=reset  InitialOutput=0
  wires:
  In/1 -> Out/1

== system uzay_vektor/ PWMA-B-C Elde edilmesi/Subsystem1/Abs Output Reset4 ==
  In : Inport
  Action : ActionPort  ActionPortLabel=elseif( u1== 4)
  Out : Outport  OutputWhenDisabled=reset  InitialOutput=0
  wires:
  In/1 -> Out/1

== system uzay_vektor/ PWMA-B-C Elde edilmesi/Subsystem1/Abs Output Reset5 ==
  In : Inport
  Action : ActionPort  ActionPortLabel=elseif(u1==5 )
  Out : Outport  OutputWhenDisabled=reset  InitialOutput=0
  wires:
  In/1 -> Out/1

== system uzay_vektor/ PWMA-B-C Elde edilmesi/Subsystem1/Abs Output Reset6 ==
  In : Inport
  Action : ActionPort  ActionPortLabel=else
  Out : Outport  OutputWhenDisabled=reset  InitialOutput=0
  wires:
  In/1 -> Out/1

== system uzay_vektor/ PWMA-B-C Elde edilmesi/Subsystem2/Abs Output Reset1 ==
  In : Inport
  Action : ActionPort  ActionPortLabel=if(u1==1)
  Out : Outport  OutputWhenDisabled=reset  InitialOutput=0
  wires:
  In/1 -> Out/1

== system uzay_vektor/ PWMA-B-C Elde edilmesi/Subsystem2/Abs Output Reset2 ==
  In : Inport
  Action : ActionPort  ActionPortLabel=elseif(u1== 2)
  Out : Outport  OutputWhenDisabled=reset  InitialOutput=0
  wires:
  In/1 -> Out/1

== system uzay_vektor/ PWMA-B-C Elde edilmesi/Subsystem2/Abs Output Reset3 ==
  In : Inport
  Action : ActionPort  ActionPortLabel=elseif(u1==3 )
  Out : Outport  OutputWhenDisabled=reset  InitialOutput=0
  wires:
  In/1 -> Out/1

== system uzay_vektor/ PWMA-B-C Elde edilmesi/Subsystem2/Abs Output Reset4 ==
  In : Inport
  Action : ActionPort  ActionPortLabel=elseif( u1== 4)
  Out : Outport  OutputWhenDisabled=reset  InitialOutput=0
  wires:
  In/1 -> Out/1

== system uzay_vektor/ PWMA-B-C Elde edilmesi/Subsystem2/Abs Output Reset5 ==
  In : Inport
  Action : ActionPort  ActionPortLabel=elseif(u1==5 )
  Out : Outport  OutputWhenDisabled=reset  InitialOutput=0
  wires:
  In/1 -> Out/1

== system uzay_vektor/ PWMA-B-C Elde edilmesi/Subsystem2/Abs Output Reset6 ==
  In : Inport
  Action : ActionPort  ActionPortLabel=else
  Out : Outport  OutputWhenDisabled=reset  InitialOutput=0
  wires:
  In/1 -> Out/1

== system uzay_vektor/ PWMA-B-C Elde edilmesi/Subsystem3/Abs Output Reset1 ==
  In : Inport
  Action : ActionPort  ActionPortLabel=if(u1==1)
  Out : Outport  OutputWhenDisabled=reset  InitialOutput=0
  wires:
  In/1 -> Out/1

== system uzay_vektor/ PWMA-B-C Elde edilmesi/Subsystem3/Abs Output Reset2 ==
  In : Inport
  Action : ActionPort  ActionPortLabel=elseif(u1== 2)
  Out : Outport  OutputWhenDisabled=reset  InitialOutput=0
  wires:
  In/1 -> Out/1

== system uzay_vektor/ PWMA-B-C Elde edilmesi/Subsystem3/Abs Output Reset3 ==
  In : Inport
  Action : ActionPort  ActionPortLabel=elseif(u1==3 )
  Out : Outport  OutputWhenDisabled=reset  InitialOutput=0
  wires:
  In/1 -> Out/1

== system uzay_vektor/ PWMA-B-C Elde edilmesi/Subsystem3/Abs Output Reset4 ==
  In : Inport
  Action : ActionPort  ActionPortLabel=elseif( u1== 4)
  Out : Outport  OutputWhenDisabled=reset  InitialOutput=0
  wires:
  In/1 -> Out/1

== system uzay_vektor/ PWMA-B-C Elde edilmesi/Subsystem3/Abs Output Reset5 ==
  In : Inport
  Action : ActionPort  ActionPortLabel=elseif(u1==5 )
  Out : Outport  OutputWhenDisabled=reset  InitialOutput=0
  wires:
  In/1 -> Out/1

== system uzay_vektor/ PWMA-B-C Elde edilmesi/Subsystem3/Abs Output Reset6 ==
  In : Inport
  Action : ActionPort  ActionPortLabel=else
  Out : Outport  OutputWhenDisabled=reset  InitialOutput=0
  wires:
  In/1 -> Out/1

== system uzay_vektor/ Çıkış Gerilimi Sİnüzoidal Dalga/Subsystem1/Abs Output Reset1 ==
  In : Inport
  Action : ActionPort  ActionPortLabel=if(u1==1)
  Out : Outport  OutputWhenDisabled=reset  InitialOutput=0
  wires:
  In/1 -> Out/1

== system uzay_vektor/ Çıkış Gerilimi Sİnüzoidal Dalga/Subsystem1/Abs Output Reset2 ==
  In : Inport
  Action : ActionPort  ActionPortLabel=elseif(u1== 2)
  Out : Outport  OutputWhenDisabled=reset  InitialOutput=0
  wires:
  In/1 -> Out/1

== system uzay_vektor/ Çıkış Gerilimi Sİnüzoidal Dalga/Subsystem1/Abs Output Reset3 ==
  In : Inport
  Action : ActionPort  ActionPortLabel=elseif(u1==3 )
  Out : Outport  OutputWhenDisabled=reset  InitialOutput=0
  wires:
  In/1 -> Out/1

== system uzay_vektor/ Çıkış Gerilimi Sİnüzoidal Dalga/Subsystem1/Abs Output Reset4 ==
  In : Inport
  Action : ActionPort  ActionPortLabel=elseif( u1== 4)
  Out : Outport  OutputWhenDisabled=reset  InitialOutput=0
  wires:
  In/1 -> Out/1

== system uzay_vektor/ Çıkış Gerilimi Sİnüzoidal Dalga/Subsystem1/Abs Output Reset5 ==
  In : Inport
  Action : ActionPort  ActionPortLabel=elseif(u1==5 )
  Out : Outport  OutputWhenDisabled=reset  InitialOutput=0
  wires:
  In/1 -> Out/1

== system uzay_vektor/ Çıkış Gerilimi Sİnüzoidal Dalga/Subsystem1/Abs Output Reset6 ==
  In : Inport
  Action : ActionPort  ActionPortLabel=else
  Out : Outport  OutputWhenDisabled=reset  InitialOutput=0
  wires:
  In/1 -> Out/1

== system uzay_vektor/ Çıkış Gerilimi Sİnüzoidal Dalga/Subsystem2/Abs Output Reset1 ==
  In : Inport
  Action : ActionPort  ActionPortLabel=if(u1==1)
  Out : Outport  OutputWhenDisabled=reset  InitialOutput=0
  wires:
  In/1 -> Out/1

== system uzay_vektor/ Çıkış Gerilimi Sİnüzoidal Dalga/Subsystem2/Abs Output Reset2 ==
  In : Inport
  Action : ActionPort  ActionPortLabel=elseif(u1== 2)
  Out : Outport  OutputWhenDisabled=reset  InitialOutput=0
  wires:
  In/1 -> Out/1

== system uzay_vektor/ Çıkış Gerilimi Sİnüzoidal Dalga/Subsystem2/Abs Output Reset3 ==
  In : Inport
  Action : ActionPort  ActionPortLabel=elseif(u1==3 )
  Out : Outport  OutputWhenDisabled=reset  InitialOutput=0
  wires:
  In/1 -> Out/1

== system uzay_vektor/ Çıkış Gerilimi Sİnüzoidal Dalga/Subsystem2/Abs Output Reset4 ==
  In : Inport
  Action : ActionPort  ActionPortLabel=elseif( u1== 4)
  Out : Outport  OutputWhenDisabled=reset  InitialOutput=0
  wires:
  In/1 -> Out/1

== system uzay_vektor/ Çıkış Gerilimi Sİnüzoidal Dalga/Subsystem2/Abs Output Reset5 ==
  In : Inport
  Action : ActionPort  ActionPortLabel=elseif(u1==5 )
  Out : Outport  OutputWhenDisabled=reset  InitialOutput=0
  wires:
  In/1 -> Out/1

== system uzay_vektor/ Çıkış Gerilimi Sİnüzoidal Dalga/Subsystem2/Abs Output Reset6 ==
  In : Inport
  Action : ActionPort  ActionPortLabel=else
  Out : Outport  OutputWhenDisabled=reset  InitialOutput=0
  wires:
  In/1 -> Out/1

== system uzay_vektor/ Çıkış Gerilimi Sİnüzoidal Dalga/Subsystem3/Abs Output Reset1 ==
  In : Inport
  Action : ActionPort  ActionPortLabel=if(u1==1)
  Out : Outport  OutputWhenDisabled=reset  InitialOutput=0
  wires:
  In/1 -> Out/1

== system uzay_vektor/ Çıkış Gerilimi Sİnüzoidal Dalga/Subsystem3/Abs Output Reset2 ==
  In : Inport
  Action : ActionPort  ActionPortLabel=elseif(u1== 2)
  Out : Outport  OutputWhenDisabled=reset  InitialOutput=0
  wires:
  In/1 -> Out/1

== system uzay_vektor/ Çıkış Gerilimi Sİnüzoidal Dalga/Subsystem3/Abs Output Reset3 ==
  In : Inport
  Action : ActionPort  ActionPortLabel=elseif(u1==3 )
  Out : Outport  OutputWhenDisabled=reset  InitialOutput=0
  wires:
  In/1 -> Out/1

== system uzay_vektor/ Çıkış Gerilimi Sİnüzoidal Dalga/Subsystem3/Abs Output Reset4 ==
  In : Inport
  Action : ActionPort  ActionPortLabel=elseif( u1== 4)
  Out : Outport  OutputWhenDisabled=reset  InitialOutput=0
  wires:
  In/1 -> Out/1

== system uzay_vektor/ Çıkış Gerilimi Sİnüzoidal Dalga/Subsystem3/Abs Output Reset5 ==
  In : Inport
  Action : ActionPort  ActionPortLabel=elseif(u1==5 )
  Out : Outport  OutputWhenDisabled=reset  InitialOutput=0
  wires:
  In/1 -> Out/1

== system uzay_vektor/ Çıkış Gerilimi Sİnüzoidal Dalga/Subsystem3/Abs Output Reset6 ==
  In : Inport
  Action : ActionPort  ActionPortLabel=else
  Out : Outport  OutputWhenDisabled=reset  InitialOutput=0
  wires:
  In/1 -> Out/1
